simulink model "APA_AEB_Version_0_1"  (R2019a)
settings: Solver=FixedStepAuto  StartTime=0.0  StopTime=2  FixedStep=0.01  RelTol=1e-3
libraries: simulink x4, dspnetwork x1, autolibshared x1
(part 1 of 3)
settings Model: DataDictionary=AEB_APA_V1.sldd  EnableAccessToBaseWorkspace=off  Creator=root  LastModifiedBy=wz527
settings DataIOCC: ReturnWorkspaceOutputs=off
settings OptimizationCC: UseDivisionForNetSlopeComputation=on  DefaultUnderspecifiedDataType=single
settings DebuggingCC: ArithmeticOperatorsInVariantConditions=warning

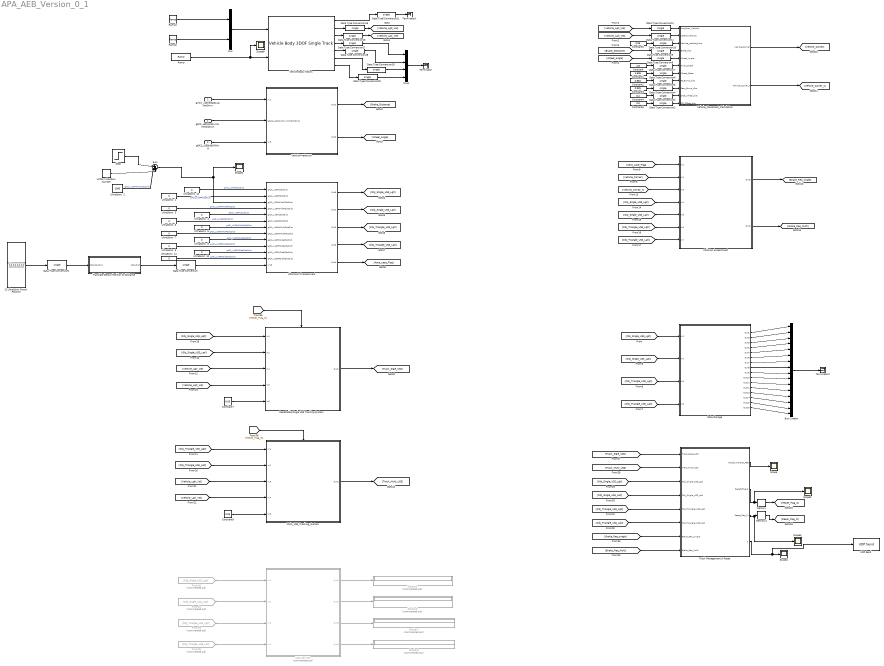
== system APA_AEB_Version_0_1 ==
  gSCS_u8RNonDrvnWhlRotlDircn : Inport
  gVCU_u16VelSpdAvgNonDrvn : Inport  Port=2
  gSAS_u16StrgWhlAng : Inport  Port=3
  12 UltraSonic Mount Position : Constant  Value=[1 1;0 0;0 0;0 0;0 0;0 0;0 0;0 0;0 0;0 0;0 0;0 0]  VectorParams1D=off
  Bus Creator : BusCreator  Inputs=16
  Collision Assessment : Subsystem
  Constant : Constant  Value=2.8
  Constant1 : Constant  Value=1.606
  Constant2 : Constant  Value=0.953
  Constant3 : Constant  Value=0.925
  Constant4 : Constant  Value=0.2
  Constant5 : Constant  Value=0.05
  Constant6 : Constant  Value=0.5
  Constant7 : Constant  Value=0.05  OutDataTypeStr=single
  Constant9 : Constant  Value=0.05  OutDataTypeStr=single
  Data Storage : Subsystem
  Data Type Conversion{,1..12,15..21} (20 alike) : DataTypeConversion  OutDataTypeStr=single
  Display{5..8} (4 alike) : Display  Commented=on
  From23 : From  Commented=on  GotoTag=Obj_Triangle_USS_Lgtl
  From24 : From  Commented=on  GotoTag=Obj_Single_USS_Latl
  From25 : From  Commented=on  GotoTag=Obj_Triangle_USS_Latl
  From26 : From  Commented=on  GotoTag=Obj_Single_USS_Lgtl
  Memory : Memory
  Memory1 : Memory
  Multi_USS_Tracking_System : Subsystem
  Mux : Mux  Inputs=2
  Mux1 : Mux
  Ramp : simulink/Sources/Ramp  slope=0.1  start=0  InitialOutput=5
  Ramp1 : simulink/Sources/Ramp  slope=1  start=0  InitialOutput=0
  Ramp2 : simulink/Sources/Ramp  slope=1  start=0  InitialOutput=0
  Resettable Single USS Tracking System : Subsystem  TreatAsAtomicUnit=on
  Scope{,1..4,9} (6 alike) : Scope
  Step : Step  After=300  SampleTime=0
  Sum : Sum  Inputs=|+++
  Terminator : Terminator
  Terminator1 : Terminator
  Terminator2 : Terminator
  Track Management & Reset : MATLAB Function  TreatAsAtomicUnit=on
  Translate Sensor Position to Distance : MATLAB Function  TreatAsAtomicUnit=on
  UDP Send : dspnetwork/UDP Send  remoteURL='192.168.101.1'  remotePort=12  localURL='0.0.0.0'  localPortSource=Automatically determine  localPort=-1  sampletime=-1  blockPlatform=[]  separateLengthPort=0
      settings: SourceProductName=Simulink
  USS Wall HMI : Subsystem  Commented=on
  "Ultarsonic Processment " : Subsystem  Tag=USS_Module  VariantControlMode=Label  Variant=on  VariantControl=Variant1  LabelModeActiveChoice=Variant1
  UltraSonic  {1,3..12} (11 alike) : Constant  Value=0  VectorParams1D=off  SampleTime=0.1
  UltraSonic  2 : Constant  Value=1000  VectorParams1D=off  SampleTime=0.1
  Uniform Random Number : UniformRandomNumber  Minimum=-100  Maximum=50  SampleTime=0.01
  Vehicle Body Motion : autolibshared/Vehicle Body 3DOF Single Track  trackMode=Dual  inputMode=External longitudinal velocity  frontSteerMode=on  rearSteerMode=off  windMode=off  muMode=off  extFMode=off  extMMode=off  extXo=off  extpsio=off  extxdoto=off  extro=off  extYo=off  extTamb=off  extydoto=off  aMode=2  NF=2  NR=2  m=2000  a=1.4  b=1.6  h=0.35  X_o=0  xdot_o=0  CalphaMode=off  sigmaMode=on  d=0  w=[1.4,1.4]  Cy_f=12e3  Cy_r=11e3  sigma_f=.1  sigma_r=.1  alpha_f_brk=[-.1 .1]  Cy_f_data=[-9e3 9e3]  alpha_r_brk=[-.1 .1]  Cy_r_data=[-9e3 9e3]  Y_o=0  ydot_o=0  Izz=4000  psi_o=0  r_o=0  Af=2  Cd=.3  Cl=.1  Cpm=.1  beta_w=[0:0.01:0.3]  Cs=[0:0.03:0.9]  Cym=[0:0.01:0.3]  Pabs=101325  Tair=273  g=9.81  mu=1  xdot_tol=.01  Fznom=5000  Fxtire_sat=7e4  Fytire_sat=7e4  longOff=0  latOff=0  vertOff=0  wrapAng=off
      settings: SourceProductName=Powertrain Blockset  SourceProductBaseCode=PW
  Vehicle Prediction : Subsystem
  Vehicle_Movement_Calculation : MATLAB Function  TreatAsAtomicUnit=on
  wires:
  gVCU_u16VelSpdAvgNonDrvn/1 -> Vehicle Prediction/1(In1)
  gSCS_u8RNonDrvnWhlRotlDircn/1 -> Vehicle Prediction/2(gSCS_u8RNonDrvnWhlRotlDircn)
  gSAS_u16StrgWhlAng/1 -> Vehicle Prediction/3(In3)
  12 UltraSonic Mount Position/1 -> Data Type Conversion1/1
  UltraSonic  12/1 -> "Ultarsonic Processment "/1(gASI_u16FLObsDist)  "gASI_u16FLObsDist"
  Vehicle Body Motion/1 -> Data Type Conversion21/1
  Vehicle Body Motion/4 -> Data Type Conversion17/1
  Vehicle Body Motion/6 -> Data Type Conversion19/1
  Vehicle Body Motion/7 -> Data Type Conversion20/1
  Vehicle Body Motion/5 -> Data Type Conversion18/1
  Mux1/1 -> Terminator/1
  Constant/1 -> Data Type Conversion7/1
  Constant1/1 -> Data Type Conversion6/1
  Constant2/1 -> Data Type Conversion5/1
  Constant3/1 -> Data Type Conversion4/1
  Constant4/1 -> Data Type Conversion3/1
  Constant5/1 -> Data Type Conversion10/1
  Constant6/1 -> Data Type Conversion2/1
  Vehicle Body Motion/2 -> Data Type Conversion15/1
  Vehicle Body Motion/3 -> Data Type Conversion16/1
  [Vehicle_Lgtl_Vel] -> Data Type Conversion12/1
  [Vehicle_Latl_Vel] -> Data Type Conversion11/1
  Vehicle Prediction/1(Out1) -> [Brake_Distance]
  Vehicle Prediction/2(Out2) -> [Wheel_Angle]
  [Brake_Distance] -> Data Type Conversion9/1
  [Wheel_Angle] -> Data Type Conversion8/1
  UltraSonic  1/1 -> "Ultarsonic Processment "/2(gASI_u16FRObsDist)  "gASI_u16FRObsDist"
  UltraSonic  3/1 -> "Ultarsonic Processment "/4(gASI_u16FrtMidRObsDist)  "gASI_u16FrtMidRObsDist"
  UltraSonic  4/1 -> "Ultarsonic Processment "/5(gASI_u16RLObsDist)  "gASI_u16RLObsDist"
  UltraSonic  5/1 -> "Ultarsonic Processment "/6(gASI_u16RRObsDist)  "gASI_u16RRObsDist"
  UltraSonic  6/1 -> "Ultarsonic Processment "/7(gASI_u16RrtMidLObsDist)  "gASI_u16RrtMidLObsDist"
  UltraSonic  7/1 -> "Ultarsonic Processment "/8(gASI_u16RrtMidRObsDist)  "gASI_u16RrtMidRObsDist"
  UltraSonic  8/1 -> "Ultarsonic Processment "/9(gASI_u16FLSideObsDist)  "gASI_u16FLSideObsDist"
  UltraSonic  9/1 -> "Ultarsonic Processment "/10(gASI_u16FRSideObsDist)  "gASI_u16FRSideObsDist"
  UltraSonic  10/1 -> "Ultarsonic Processment "/11(gASI_u16RLSideObsDist)  "gASI_u16RLSideObsDist"
  UltraSonic  11/1 -> "Ultarsonic Processment "/12(gASI_u16RRSideObsDist)  "gASI_u16RRSideObsDist"
  Translate Sensor Position to Distance/1(USS_Dist) -> Data Type Conversion/1
  "Ultarsonic Processment "/1(Out6) -> [Obj_Single_USS_Lgtl]
  "Ultarsonic Processment "/2(Out1) -> [Obj_Single_USS_Latl]
  "Ultarsonic Processment "/3(Out2) -> [Obj_Triangle_USS_Lgtl]
  "Ultarsonic Processment "/4(Out3) -> [Obj_Triangle_USS_Latl]
  Vehicle_Movement_Calculation/1(Vehicle_Corner) -> [Vehicle_Corner]
  Vehicle_Movement_Calculation/2(Vehicle_Corner_t) -> [Vehicle_Corner_t]
  [Obj_Single_USS_Lgtl] -> Data Storage/1(In2)
  [Obj_Single_USS_Latl] -> Data Storage/2(In4)
  [Obj_Triangle_USS_Lgtl] -> Data Storage/3(In5)
  [Obj_Triangle_USS_Latl] -> Data Storage/4(In6)
  "Ultarsonic Processment "/5(Out4) -> [Aera_case_Flag]
  [Aera_case_Flag] -> Collision Assessment/1(In1)
  [Vehicle_Corner] -> Collision Assessment/2(In2)
  [Vehicle_Corner_t] -> Collision Assessment/3(In3)
  [Obj_Single_USS_Lgtl] -> Collision Assessment/4(In4)
  [Obj_Single_USS_Latl] -> Collision Assessment/5(In5)
  [Obj_Triangle_USS_Lgtl] -> Collision Assessment/6(In6)
  [Obj_Triangle_USS_Latl] -> Collision Assessment/7(In7)
  Data Storage/1(Out1) -> Bus Creator/1
  Data Storage/2(Out3) -> Bus Creator/2
  Data Storage/3(Out5) -> Bus Creator/3
  Data Storage/4(Out2) -> Bus Creator/4
  Data Storage/5(Out4) -> Bus Creator/5
  Data Storage/6(Out6) -> Bus Creator/6
  Data Storage/7(Out7) -> Bus Creator/7
  Data Storage/8(Out8) -> Bus Creator/8
  Data Storage/9(Out9) -> Bus Creator/9
  Data Storage/10(Out10) -> Bus Creator/10
  Data Storage/11(Out11) -> Bus Creator/11
  Data Storage/12(Out12) -> Bus Creator/12
  Data Storage/13(Out13) -> Bus Creator/13
  Data Storage/14(Out14) -> Bus Creator/14
  Data Storage/15(Out15) -> Bus Creator/15
  Data Storage/16(Out16) -> Bus Creator/16
  Bus Creator/1 -> Terminator2/1
  [Obj_Single_USS_Lgtl] -> Resettable Single USS Tracking System/1(In1)
  [Obj_Single_USS_Latl] -> Resettable Single USS Tracking System/2(In2)
  [Vehicle_Lgtl_Vel] -> Resettable Single USS Tracking System/3(In4)
  [Vehicle_Latl_Vel] -> Resettable Single USS Tracking System/4(In5)
  Constant7/1 -> Resettable Single USS Tracking System/5(In6)
  Resettable Single USS Tracking System/1(Out1) -> [Track_Sigle_USS]
  Collision Assessment/1(Out3) -> [Brake_Req_single]
  Collision Assessment/2(Out1) -> [Brake_Req_Multi]
  UltraSonic  2/1 -> Sum/2  "gASI_u16FrtMidLObsDist"
  Sum/1 -> "Ultarsonic Processment "/3(gASI_u16FrtMidLObsDist), Scope1/1
  [Obj_Triangle_USS_Lgtl] -> Multi_USS_Tracking_System/1(In1)
  [Obj_Triangle_USS_Latl] -> Multi_USS_Tracking_System/2(In2)
  [Vehicle_Lgtl_Vel] -> Multi_USS_Tracking_System/3(In3)
  [Vehicle_Latl_Vel] -> Multi_USS_Tracking_System/4(In4)
  Constant9/1 -> Multi_USS_Tracking_System/5(In5)
  Multi_USS_Tracking_System/1(Out1) -> [Track_Multi_USS]
  From26/1 -> USS Wall HMI/1(In1)
  From24/1 -> USS Wall HMI/2(In2)
  From23/1 -> USS Wall HMI/3(In3)
  From25/1 -> USS Wall HMI/4(In4)
  USS Wall HMI/1(Out1) -> Display5/1
  USS Wall HMI/2(Out2) -> Display6/1
  USS Wall HMI/3(Out3) -> Display7/1
  USS Wall HMI/4(Out4) -> Display8/1
  [Track_Sigle_USS] -> Track Management & Reset/1(Track_Sigle_USS)
  [Track_Multi_USS] -> Track Management & Reset/2(Track_Multi_USS)
  [Obj_Single_USS_Lgtl] -> Track Management & Reset/3(Obj_Single_USS_Lgtl)
  [Obj_Single_USS_Latl] -> Track Management & Reset/4(Obj_Single_USS_Latl)
  [Obj_Triangle_USS_Lgtl] -> Track Management & Reset/5(Obj_Triangle_USS_Lgtl)
  [Obj_Triangle_USS_Latl] -> Track Management & Reset/6(Obj_Triangle_USS_Latl)
  [Brake_Req_single] -> Track Management & Reset/7(Brake_Req_single)
  [Brake_Req_Multi] -> Track Management & Reset/8(Brake_Req_Multi)
  Step/1 -> Sum/1
  Uniform Random Number/1 -> Sum/3
  Track Management & Reset/1(Global_Tracker_AEB) -> Scope/1
  Track Management & Reset/2(Reset_Flag_S) -> Scope2/1, Memory/1
  Track Management & Reset/3(Reset_Flag_M) -> Scope3/1, Memory1/1
  [Reset_Flag_S] -> Resettable Single USS Tracking System/Reset
  [Reset_Flag_M] -> Multi_USS_Tracking_System/Reset
  Memory/1 -> [Reset_Flag_S]
  Memory1/1 -> [Reset_Flag_M]
  Track Management & Reset/4(c) -> UDP Send/1, Scope4/1
  Data Type Conversion/1 -> "Ultarsonic Processment "/13(In13)
  Data Type Conversion1/1 -> Translate Sensor Position to Distance/1(USS_Position)
  Data Type Conversion2/1 -> Vehicle_Movement_Calculation/11(CG_Offset_dist)
  Data Type Conversion3/1 -> Vehicle_Movement_Calculation/10(Side_wheel_dist)
  Data Type Conversion4/1 -> Vehicle_Movement_Calculation/9(Rear_Bump_dist)
  Data Type Conversion5/1 -> Vehicle_Movement_Calculation/8(Frt_Bump_dist)
  Data Type Conversion6/1 -> Vehicle_Movement_Calculation/7(Wheel_Base)
  Data Type Conversion7/1 -> Vehicle_Movement_Calculation/6(Axle_Length)
  Data Type Conversion8/1 -> Vehicle_Movement_Calculation/5(Wheel_Angle)
  Data Type Conversion9/1 -> Vehicle_Movement_Calculation/4(Brake_dist)
  Data Type Conversion10/1 -> Vehicle_Movement_Calculation/3(Vehicle_predict_time)
  Data Type Conversion11/1 -> Vehicle_Movement_Calculation/2(Lateral_Velocity)
  Data Type Conversion12/1 -> Vehicle_Movement_Calculation/1(Longitual_Velocity)
  Mux/1 -> Vehicle Body Motion/1
  Data Type Conversion15/1 -> [Vehicle_Lgtl_Vel]
  Data Type Conversion16/1 -> [Vehicle_Latl_Vel]
  Data Type Conversion17/1 -> Mux1/1
  Data Type Conversion18/1 -> Mux1/2
  Data Type Conversion19/1 -> Mux1/3
  Data Type Conversion20/1 -> Mux1/4
  Data Type Conversion21/1 -> Terminator1/1
  Ramp1/1 -> Mux/1
  Ramp2/1 -> Mux/2
  Ramp/1 -> Scope9/1, Vehicle Body Motion/2

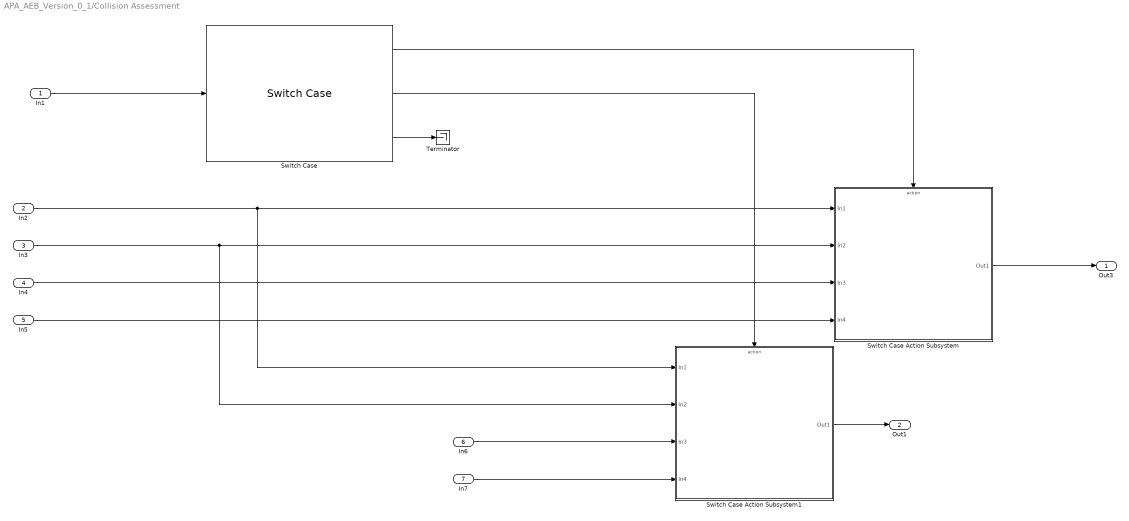
== system APA_AEB_Version_0_1/Collision Assessment ==
  In1 : Inport
  In2 : Inport  Port=2
  In3 : Inport  Port=3
  In4 : Inport  Port=4
  In5 : Inport  Port=5
  In6 : Inport  Port=6
  In7 : Inport  Port=7
  Switch Case : SwitchCase  CaseConditions={[1,2,3,4,5,6,7,8,9,10,11,12],[14,15,16,20,21,22]}
  Switch Case Action Subsystem : Subsystem  TreatAsAtomicUnit=on
  Switch Case Action Subsystem1 : Subsystem  TreatAsAtomicUnit=on
  Terminator : Terminator
  Out3 : Outport
  Out1 : Outport  Port=2
  wires:
  Switch Case Action Subsystem/1(Out1) -> Out3/1
  Switch Case/2 -> Switch Case Action Subsystem1/Action
  In1/1 -> Switch Case/1
  In2/1 -> Switch Case Action Subsystem1/1(In1), Switch Case Action Subsystem/1(In1)
  In4/1 -> Switch Case Action Subsystem/3(In3)
  In3/1 -> Switch Case Action Subsystem1/2(In2), Switch Case Action Subsystem/2(In2)
  Switch Case/3 -> Terminator/1
  In5/1 -> Switch Case Action Subsystem/4(In4)
  Switch Case/1 -> Switch Case Action Subsystem/Action
  In6/1 -> Switch Case Action Subsystem1/3(In3)
  In7/1 -> Switch Case Action Subsystem1/4(In4)
  Switch Case Action Subsystem1/1(Out1) -> Out1/1

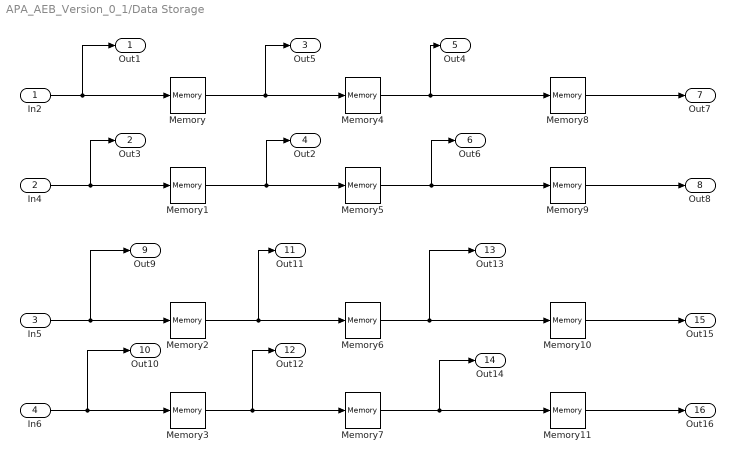
== system APA_AEB_Version_0_1/Data Storage ==
  In2 : Inport
  In4 : Inport  Port=2
  In5 : Inport  Port=3
  In6 : Inport  Port=4
  Memory{,1..11} (12 alike) : Memory
  Out1 : Outport
  Out3 : Outport  Port=2
  Out5 : Outport  Port=3
  Out2 : Outport  Port=4
  Out4 : Outport  Port=5
  Out6 : Outport  Port=6
  Out7 : Outport  Port=7
  Out8 : Outport  Port=8
  Out9 : Outport  Port=9
  Out10 : Outport  Port=10
  Out11 : Outport  Port=11
  Out12 : Outport  Port=12
  Out13 : Outport  Port=13
  Out14 : Outport  Port=14
  Out15 : Outport  Port=15
  Out16 : Outport  Port=16
  wires:
  Memory3/1 -> Out12/1, Memory7/1
  Memory2/1 -> Out11/1, Memory6/1
  Memory7/1 -> Out14/1, Memory11/1
  Memory6/1 -> Out13/1, Memory10/1
  In5/1 -> Out9/1, Memory2/1
  In4/1 -> Out3/1, Memory1/1
  Memory/1 -> Out5/1, Memory4/1
  Memory1/1 -> Memory5/1, Out2/1
  In6/1 -> Out10/1, Memory3/1
  Memory4/1 -> Out4/1, Memory8/1
  Memory5/1 -> Memory9/1, Out6/1
  Memory8/1 -> Out7/1
  Memory9/1 -> Out8/1
  In2/1 -> Out1/1, Memory/1
  Memory10/1 -> Out15/1
  Memory11/1 -> Out16/1

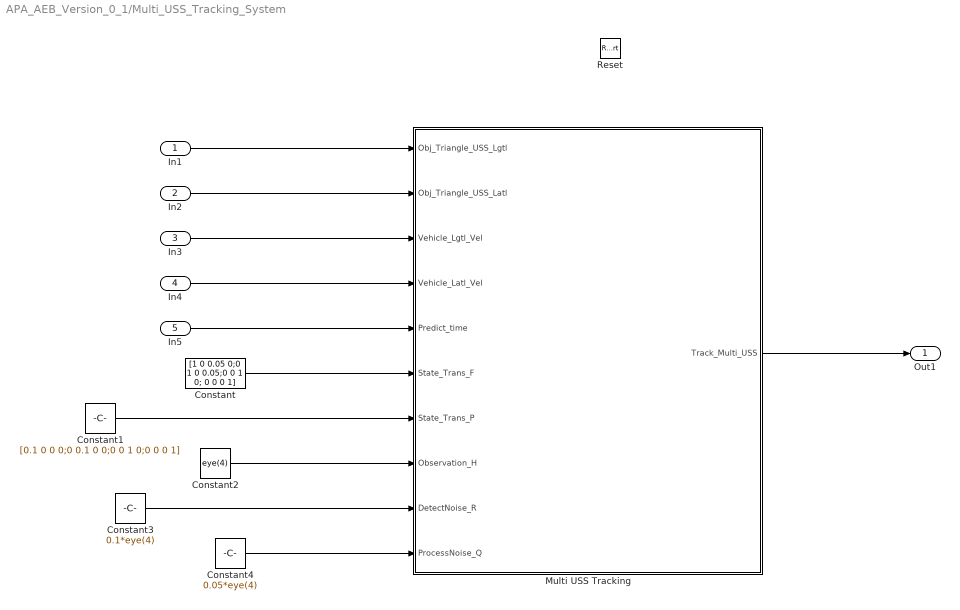
== system APA_AEB_Version_0_1/Multi_USS_Tracking_System ==
  In1 : Inport
  In2 : Inport  Port=2
  In3 : Inport  Port=3
  In4 : Inport  Port=4
  In5 : Inport  Port=5
  Reset : ResetPort  DisableCoverage=on  ResetTriggerType=level hold
  Constant : Constant  Value=[1 0 0.05 0;0 1 0 0.05;0 0 1 0; 0 0 0 1]  OutDataTypeStr=single
  Constant1 : Constant  Value=[0.1 0 0 0;0 0.1 0 0;0 0 1 0;0 0 0 1]  OutDataTypeStr=single
  Constant2 : Constant  Value=eye(4)  OutDataTypeStr=single
  Constant3 : Constant  Value=0.1*eye(4)  OutDataTypeStr=single
  Constant4 : Constant  Value=0.05*eye(4)  OutDataTypeStr=single
  Multi USS Tracking : MATLAB Function  TreatAsAtomicUnit=on
  Out1 : Outport
  wires:
  In4/1 -> Multi USS Tracking/4(Vehicle_Latl_Vel)
  Multi USS Tracking/1(Track_Multi_USS) -> Out1/1
  Constant4/1 -> Multi USS Tracking/10(ProcessNoise_Q)
  In5/1 -> Multi USS Tracking/5(Predict_time)
  Constant1/1 -> Multi USS Tracking/7(State_Trans_P)
  Constant2/1 -> Multi USS Tracking/8(Observation_H)
  Constant/1 -> Multi USS Tracking/6(State_Trans_F)
  In3/1 -> Multi USS Tracking/3(Vehicle_Lgtl_Vel)
  Constant3/1 -> Multi USS Tracking/9(DetectNoise_R)
  In1/1 -> Multi USS Tracking/1(Obj_Triangle_USS_Lgtl)
  In2/1 -> Multi USS Tracking/2(Obj_Triangle_USS_Latl)

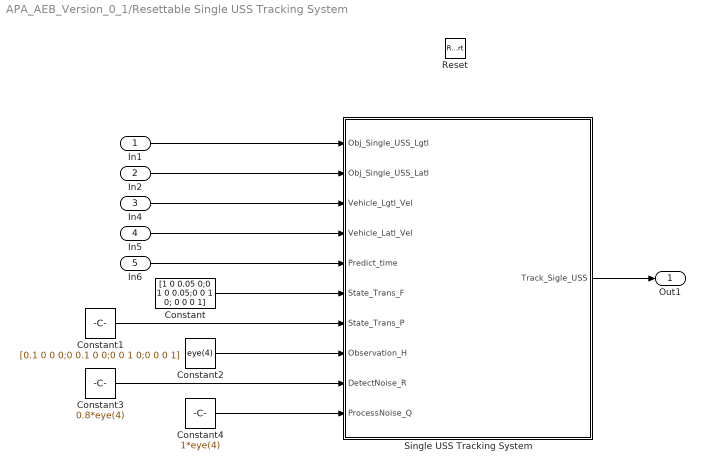
== system APA_AEB_Version_0_1/Resettable Single USS Tracking System ==
  In1 : Inport
  In2 : Inport  Port=2
  In4 : Inport  Port=3
  In5 : Inport  Port=4
  In6 : Inport  Port=5
  Reset : ResetPort  DisableCoverage=on  ResetTriggerType=level hold
  Constant : Constant  Value=[1 0 0.05 0;0 1 0 0.05;0 0 1 0; 0 0 0 1]  OutDataTypeStr=single
  Constant1 : Constant  Value=[0.1 0 0 0;0 0.1 0 0;0 0 1 0;0 0 0 1]  OutDataTypeStr=single
  Constant2 : Constant  Value=eye(4)  OutDataTypeStr=single
  Constant3 : Constant  Value=0.8*eye(4)  OutDataTypeStr=single
  Constant4 : Constant  Value=1*eye(4)  OutDataTypeStr=single
  Single USS Tracking System : MATLAB Function  TreatAsAtomicUnit=on
  Out1 : Outport
  wires:
  Single USS Tracking System/1(Track_Sigle_USS) -> Out1/1
  In1/1 -> Single USS Tracking System/1(Obj_Single_USS_Lgtl)
  In4/1 -> Single USS Tracking System/3(Vehicle_Lgtl_Vel)
  In5/1 -> Single USS Tracking System/4(Vehicle_Latl_Vel)
  In2/1 -> Single USS Tracking System/2(Obj_Single_USS_Latl)
  In6/1 -> Single USS Tracking System/5(Predict_time)
  Constant/1 -> Single USS Tracking System/6(State_Trans_F)
  Constant1/1 -> Single USS Tracking System/7(State_Trans_P)
  Constant2/1 -> Single USS Tracking System/8(Observation_H)
  Constant3/1 -> Single USS Tracking System/9(DetectNoise_R)
  Constant4/1 -> Single USS Tracking System/10(ProcessNoise_Q)

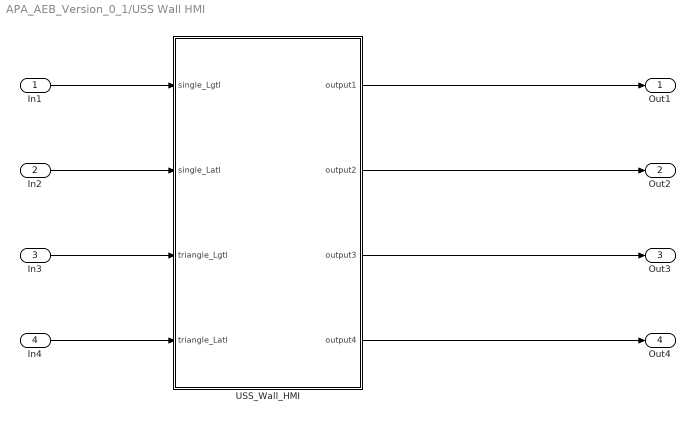
== system APA_AEB_Version_0_1/USS Wall HMI ==
  In1 : Inport
  In2 : Inport  Port=2
  In3 : Inport  Port=3
  In4 : Inport  Port=4
  USS_Wall_HMI : MATLAB Function  TreatAsAtomicUnit=on
  Out1 : Outport
  Out2 : Outport  Port=2
  Out3 : Outport  Port=3
  Out4 : Outport  Port=4
  wires:
  In2/1 -> USS_Wall_HMI/2(single_Latl)
  USS_Wall_HMI/1(output1) -> Out1/1
  In3/1 -> USS_Wall_HMI/3(triangle_Lgtl)
  USS_Wall_HMI/2(output2) -> Out2/1
  USS_Wall_HMI/3(output3) -> Out3/1
  In1/1 -> USS_Wall_HMI/1(single_Lgtl)
  In4/1 -> USS_Wall_HMI/4(triangle_Latl)
  USS_Wall_HMI/4(output4) -> Out4/1

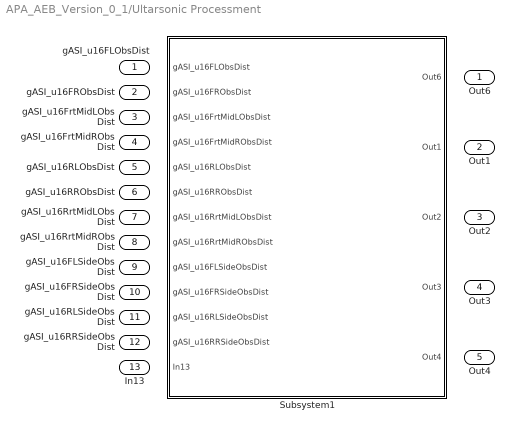
== system APA_AEB_Version_0_1/Ultarsonic Processment  ==
  gASI_u16FLObsDist : Inport
  gASI_u16FRObsDist : Inport  Port=2
  gASI_u16FrtMidLObsDist : Inport  Port=3
  gASI_u16FrtMidRObsDist : Inport  Port=4
  gASI_u16RLObsDist : Inport  Port=5
  gASI_u16RRObsDist : Inport  Port=6
  gASI_u16RrtMidLObsDist : Inport  Port=7
  gASI_u16RrtMidRObsDist : Inport  Port=8
  gASI_u16FLSideObsDist : Inport  Port=9
  gASI_u16FRSideObsDist : Inport  Port=10
  gASI_u16RLSideObsDist : Inport  Port=11
  gASI_u16RRSideObsDist : Inport  Port=12
  In13 : Inport  Port=13
  Subsystem1 : Subsystem  VariantControlMode=Label  Variant=on  VariantControl=Variant1  LabelModeActiveChoice=Variant1
  Out6 : Outport
  Out1 : Outport  Port=2
  Out2 : Outport  Port=3
  Out3 : Outport  Port=4
  Out4 : Outport  Port=5

== system APA_AEB_Version_0_1/Vehicle Prediction ==
  In1 : Inport
  gSCS_u8RNonDrvnWhlRotlDircn : Inport  Port=2
  In3 : Inport  Port=3
  Subsystem : Subsystem
  Subsystem1 : Subsystem
  Out1 : Outport
  Out2 : Outport  Port=2
  wires:
  In1/1 -> Subsystem/1(In1)
  gSCS_u8RNonDrvnWhlRotlDircn/1 -> Subsystem/2(gSCS_u8RNonDrvnWhlRotlDircn)
  Subsystem/1(Out1) -> Out1/1
  In3/1 -> Subsystem1/1(In1)
  Subsystem1/1(Out1) -> Out2/1

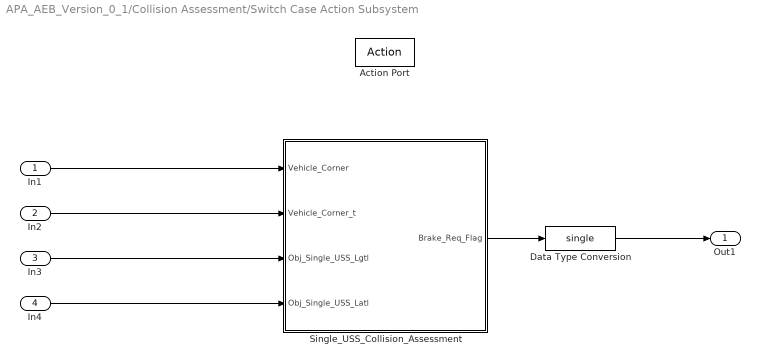
== system APA_AEB_Version_0_1/Collision Assessment/Switch Case Action Subsystem ==
  In1 : Inport
  In2 : Inport  Port=2
  In3 : Inport  Port=3
  In4 : Inport  Port=4
  Action Port : ActionPort  ActionPortLabel=case [ 1 2 3 4 5 6 7 8 9 10 11 12 ]:
  Data Type Conversion : DataTypeConversion  OutDataTypeStr=single
  Single_USS_Collision_Assessment : MATLAB Function  TreatAsAtomicUnit=on
  Out1 : Outport
  wires:
  In1/1 -> Single_USS_Collision_Assessment/1(Vehicle_Corner)
  In2/1 -> Single_USS_Collision_Assessment/2(Vehicle_Corner_t)
  In3/1 -> Single_USS_Collision_Assessment/3(Obj_Single_USS_Lgtl)
  In4/1 -> Single_USS_Collision_Assessment/4(Obj_Single_USS_Latl)
  Single_USS_Collision_Assessment/1(Brake_Req_Flag) -> Data Type Conversion/1
  Data Type Conversion/1 -> Out1/1

== system APA_AEB_Version_0_1/Collision Assessment/Switch Case Action Subsystem1 ==
  In1 : Inport
  In2 : Inport  Port=2
  In3 : Inport  Port=3
  In4 : Inport  Port=4
  Action Port : ActionPort  ActionPortLabel=case [ 14 15 16 20 21 22 ]:
  Multi_USS_Collision_Assessment : MATLAB Function  TreatAsAtomicUnit=on
  Out1 : Outport
  wires:
  Multi_USS_Collision_Assessment/1(Brake_Req_Flag) -> Out1/1
  In4/1 -> Multi_USS_Collision_Assessment/4(Obj_Triangle_USS_Latl)
  In3/1 -> Multi_USS_Collision_Assessment/3(Obj_Triangle_USS_Lgtl)
  In2/1 -> Multi_USS_Collision_Assessment/2(Vehicle_Corner_t)
  In1/1 -> Multi_USS_Collision_Assessment/1(Vehicle_Corner)

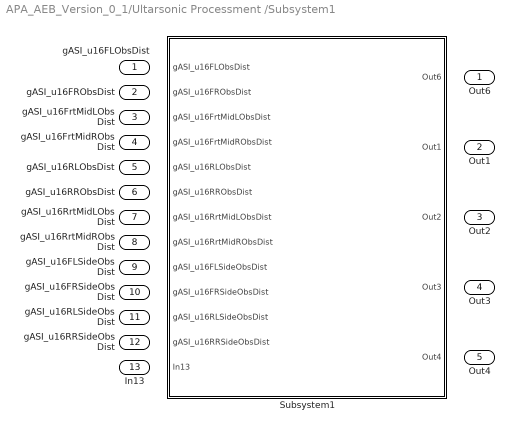
== system APA_AEB_Version_0_1/Ultarsonic Processment /Subsystem1 ==
  gASI_u16FLObsDist : Inport
  gASI_u16FRObsDist : Inport  Port=2
  gASI_u16FrtMidLObsDist : Inport  Port=3
  gASI_u16FrtMidRObsDist : Inport  Port=4
  gASI_u16RLObsDist : Inport  Port=5
  gASI_u16RRObsDist : Inport  Port=6
  gASI_u16RrtMidLObsDist : Inport  Port=7
  gASI_u16RrtMidRObsDist : Inport  Port=8
  gASI_u16FLSideObsDist : Inport  Port=9
  gASI_u16FRSideObsDist : Inport  Port=10
  gASI_u16RLSideObsDist : Inport  Port=11
  gASI_u16RRSideObsDist : Inport  Port=12
  In13 : Inport  Port=13
  Subsystem1 : Subsystem  VariantControl=Variant1
  Out6 : Outport
  Out1 : Outport  Port=2
  Out2 : Outport  Port=3
  Out3 : Outport  Port=4
  Out4 : Outport  Port=5

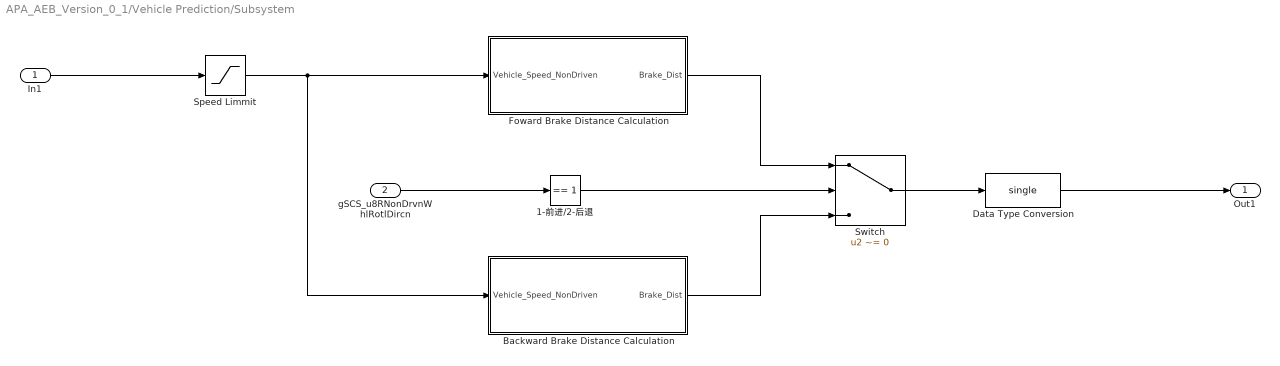
== system APA_AEB_Version_0_1/Vehicle Prediction/Subsystem ==
  In1 : Inport
  gSCS_u8RNonDrvnWhlRotlDircn : Inport  Port=2
  1-前进/2-后退 : simulink/Logic and Bit Operations/Compare To Constant  relop===  const=1  OutDataTypeStr=boolean
  Backward Brake Distance Calculation : MATLAB Function  TreatAsAtomicUnit=on
  Data Type Conversion : DataTypeConversion  OutDataTypeStr=single
  Foward Brake Distance Calculation : MATLAB Function  TreatAsAtomicUnit=on
  Speed Limmit : Saturate  UpperLimit=6  LowerLimit=0
  Switch : Switch  Criteria=u2 ~= 0
  Out1 : Outport
  wires:
  Backward Brake Distance Calculation/1(Brake_Dist) -> Switch/3
  Speed Limmit/1 -> Backward Brake Distance Calculation/1(Vehicle_Speed_NonDriven), Foward Brake Distance Calculation/1(Vehicle_Speed_NonDriven)
  Data Type Conversion/1 -> Out1/1
  Foward Brake Distance Calculation/1(Brake_Dist) -> Switch/1
  1-前进/2-后退/1 -> Switch/2
  Switch/1 -> Data Type Conversion/1
  gSCS_u8RNonDrvnWhlRotlDircn/1 -> 1-前进/2-后退/1
  In1/1 -> Speed Limmit/1

== system APA_AEB_Version_0_1/Vehicle Prediction/Subsystem1 ==
  In1 : Inport
  Data Type Conversion1 : DataTypeConversion  OutDataTypeStr=single
  Data Type Conversion3 : DataTypeConversion  OutDataTypeStr=single
  Steer Angle To Wheel Angle : MATLAB Function  TreatAsAtomicUnit=on
  Out1 : Outport
  wires:
  Data Type Conversion3/1 -> Steer Angle To Wheel Angle/1(Steer_Angle)
  Steer Angle To Wheel Angle/1(Wheel_Angle) -> Data Type Conversion1/1
  In1/1 -> Data Type Conversion3/1
  Data Type Conversion1/1 -> Out1/1

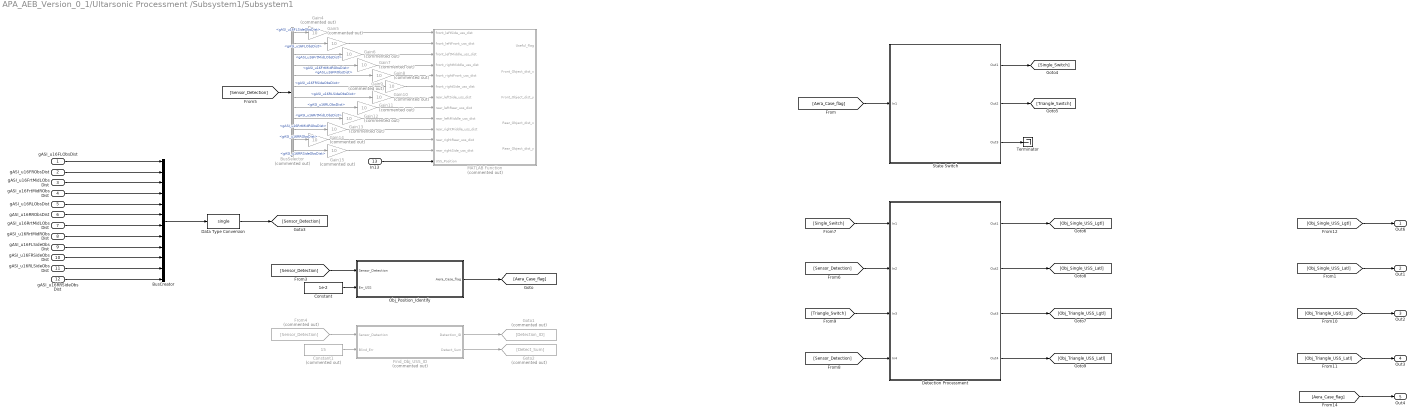
== system APA_AEB_Version_0_1/Ultarsonic Processment /Subsystem1/Subsystem1 ==
  gASI_u16FLObsDist : Inport
  gASI_u16FRObsDist : Inport  Port=2
  gASI_u16FrtMidLObsDist : Inport  Port=3
  gASI_u16FrtMidRObsDist : Inport  Port=4
  gASI_u16RLObsDist : Inport  Port=5
  gASI_u16RRObsDist : Inport  Port=6
  gASI_u16RrtMidLObsDist : Inport  Port=7
  gASI_u16RrtMidRObsDist : Inport  Port=8
  gASI_u16FLSideObsDist : Inport  Port=9
  gASI_u16FRSideObsDist : Inport  Port=10
  gASI_u16RLSideObsDist : Inport  Port=11
  gASI_u16RRSideObsDist : Inport  Port=12
  In13 : Inport  Port=13
  BusCreator : BusCreator  Inputs=12
  BusSelector : BusSelector  Commented=on  OutputSignals=gASI_u16FLSideObsDist,gASI_u16FLObsDist,gASI_u16FrtMidLObsDist,gASI_u16FrtMidRObsDist,gASI_u16FRObsDist,gASI_u16FRSideObsDist,gASI_u16RLSideObsDist,gASI_u16RLObsDist,gASI_u16RrtMidLObsDist,gASI_u16RrtMidRObsDist,gASI_u16RRObsDist,gASI_u16RRSideObsDist
  Constant : Constant  Value=1e-2  OutDataTypeStr=single
  Constant1 : Constant  Commented=on  Value=15
  Data Type Conversion : DataTypeConversion  OutDataTypeStr=single
  Detection Processment : Subsystem
  Find_Obj_USS_ID : MATLAB Function  Commented=on  TreatAsAtomicUnit=on
  From4 : From  Commented=on  GotoTag=Sensor_Detection
  Gain{4..15} (12 alike) : Gain  Commented=on  Gain=10  OutDataTypeStr=Inherit: Same as input
  Goto1 : Goto  Commented=on  GotoTag=Detection_ID
  Goto2 : Goto  Commented=on  GotoTag=Detect_Sum
  MATLAB Function : MATLAB Function  Commented=on  TreatAsAtomicUnit=on
  Obj_Position_Identify : MATLAB Function  TreatAsAtomicUnit=on
  State Switch : Subsystem
  Terminator : Terminator
  Out6 : Outport
  Out1 : Outport  Port=2
  Out2 : Outport  Port=3
  Out3 : Outport  Port=4
  Out4 : Outport  Port=5
  wires:
  BusSelector/5 -> Gain8/1  "<gASI_u16FRObsDist>"
  BusCreator/1 -> Data Type Conversion/1
  BusSelector/1 -> Gain4/1  "<gASI_u16FLSideObsDist>"
  gASI_u16RRObsDist/1 -> BusCreator/6
  BusSelector/10 -> Gain13/1  "<gASI_u16RrtMidRObsDist>"
  BusSelector/4 -> Gain7/1  "<gASI_u16FrtMidRObsDist>"
  Gain13/1 -> MATLAB Function/10(rear_rightMiddle_uss_dist)
  BusSelector/3 -> Gain6/1  "<gASI_u16FrtMidLObsDist>"
  BusSelector/11 -> Gain14/1  "<gASI_u16RRObsDist>"
  gASI_u16FRSideObsDist/1 -> BusCreator/10
  BusSelector/12 -> Gain15/1  "<gASI_u16RRSideObsDist>"
  Gain9/1 -> MATLAB Function/6(front_rightSide_uss_dist)
  Gain10/1 -> MATLAB Function/7(rear_leftSide_uss_dist)
  BusSelector/8 -> Gain11/1  "<gASI_u16RLObsDist>"
  Gain7/1 -> MATLAB Function/4(front_rightMiddle_uss_dist)
  BusSelector/6 -> Gain9/1  "<gASI_u16FRSideObsDist>"
  gASI_u16FrtMidRObsDist/1 -> BusCreator/4
  Gain5/1 -> MATLAB Function/2(front_leftFront_uss_dist)
  Gain11/1 -> MATLAB Function/8(rear_leftRear_uss_dist)
  Gain4/1 -> MATLAB Function/1(front_leftSide_uss_dist)
  In13/1 -> MATLAB Function/13(USS_Position)
  gASI_u16FRObsDist/1 -> BusCreator/2
  Gain12/1 -> MATLAB Function/9(rear_leftMiddle_uss_dist)
  Gain8/1 -> MATLAB Function/5(front_rightFront_uss_dist)
  gASI_u16RRSideObsDist/1 -> BusCreator/12
  Gain14/1 -> MATLAB Function/11(rear_rightRear_uss_dist)
  Gain6/1 -> MATLAB Function/3(front_leftMiddle_uss_dist)
  gASI_u16RrtMidLObsDist/1 -> BusCreator/7
  Gain15/1 -> MATLAB Function/12(rear_rightSide_uss_dist)
  BusSelector/2 -> Gain5/1  "<gASI_u16FLObsDist>"
  BusSelector/7 -> Gain10/1  "<gASI_u16RLSideObsDist>"
  gASI_u16RLSideObsDist/1 -> BusCreator/11
  BusSelector/9 -> Gain12/1  "<gASI_u16RrtMidLObsDist>"
  gASI_u16FLSideObsDist/1 -> BusCreator/9
  gASI_u16RLObsDist/1 -> BusCreator/5
  gASI_u16RrtMidRObsDist/1 -> BusCreator/8
  gASI_u16FLObsDist/1 -> BusCreator/1
  gASI_u16FrtMidLObsDist/1 -> BusCreator/3
  Constant/1 -> Obj_Position_Identify/2(Err_USS)
  Constant1/1 -> Find_Obj_USS_ID/2(Blind_Err)
  Obj_Position_Identify/1(Aera_Case_flag) -> [Aera_Case_flag]
  Find_Obj_USS_ID/2(Detect_Sum) -> Goto2/1
  Find_Obj_USS_ID/1(Detection_ID) -> Goto1/1
  [Sensor_Detection] -> Obj_Position_Identify/1(Sensor_Detection)
  From4/1 -> Find_Obj_USS_ID/1(Sensor_Detection)
  [Sensor_Detection] -> BusSelector/1
  [Single_Switch] -> Detection Processment/1(In1)
  [Sensor_Detection] -> Detection Processment/2(In2)
  [Triangle_Switch] -> Detection Processment/3(In3)
  [Sensor_Detection] -> Detection Processment/4(In4)
  Detection Processment/3(Out3) -> [Obj_Triangle_USS_Lgtl]
  [Aera_Case_flag] -> State Switch/1(In1)
  State Switch/1(Out1) -> [Single_Switch]
  State Switch/2(Out2) -> [Triangle_Switch]
  Detection Processment/2(Out2) -> [Obj_Single_USS_Latl]
  Detection Processment/4(Out4) -> [Obj_Triangle_USS_Latl]
  Detection Processment/1(Out1) -> [Obj_Single_USS_Lgtl]
  [Obj_Single_USS_Lgtl] -> Out6/1
  [Obj_Single_USS_Latl] -> Out1/1
  [Obj_Triangle_USS_Lgtl] -> Out2/1
  [Obj_Triangle_USS_Latl] -> Out3/1
  State Switch/3(Out3) -> Terminator/1
  [Aera_Case_flag] -> Out4/1
  Data Type Conversion/1 -> [Sensor_Detection]

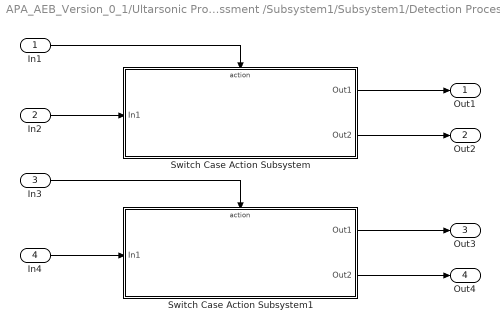
== system APA_AEB_Version_0_1/Ultarsonic Processment /Subsystem1/Subsystem1/Detection Processment ==
  In1 : Inport
  In2 : Inport  Port=2
  In3 : Inport  Port=3
  In4 : Inport  Port=4
  Switch Case Action Subsystem : Subsystem  TreatAsAtomicUnit=on
  Switch Case Action Subsystem1 : Subsystem  TreatAsAtomicUnit=on
  Out1 : Outport
  Out2 : Outport  Port=2
  Out3 : Outport  Port=3
  Out4 : Outport  Port=4
  wires:
  In3/1 -> Switch Case Action Subsystem1/Action
  In4/1 -> Switch Case Action Subsystem1/1(In1)
  In1/1 -> Switch Case Action Subsystem/Action
  Switch Case Action Subsystem1/1(Out1) -> Out3/1
  In2/1 -> Switch Case Action Subsystem/1(In1)
  Switch Case Action Subsystem/1(Out1) -> Out1/1
  Switch Case Action Subsystem/2(Out2) -> Out2/1
  Switch Case Action Subsystem1/2(Out2) -> Out4/1

== system APA_AEB_Version_0_1/Ultarsonic Processment /Subsystem1/Subsystem1/State Switch ==
  In1 : Inport
  Switch Case : SwitchCase  CaseConditions={[1,2,3,4,5,6,7,8,9,10,11,12],[14,15,16,20,21,22]}
  Out1 : Outport
  Out2 : Outport  Port=2
  Out3 : Outport  Port=3
  wires:
  Switch Case/3 -> Out3/1
  In1/1 -> Switch Case/1
  Switch Case/2 -> Out2/1
  Switch Case/1 -> Out1/1

== system APA_AEB_Version_0_1/Ultarsonic Processment /Subsystem1/Subsystem1/Detection Processment/Switch Case Action Subsystem ==
  In1 : Inport
  Action Port : ActionPort  ActionPortLabel=case [ 1 2 3 4 5 6 7 8 9 10 11 12 ]:
  MATLAB Function : MATLAB Function  TreatAsAtomicUnit=on
  Out1 : Outport
  Out2 : Outport  Port=2
  wires:
  In1/1 -> MATLAB Function/1(Sensor_Detection)
  MATLAB Function/1(Longitudial_Dist) -> Out1/1
  MATLAB Function/2(Lateral_Dist) -> Out2/1

== system APA_AEB_Version_0_1/Ultarsonic Processment /Subsystem1/Subsystem1/Detection Processment/Switch Case Action Subsystem1 ==
  In1 : Inport
  Action Port : ActionPort  ActionPortLabel=case [ 14 15 16 20 21 22 ]:
  MATLAB Function : MATLAB Function  TreatAsAtomicUnit=on
  Out1 : Outport
  Out2 : Outport  Port=2
  wires:
  In1/1 -> MATLAB Function/1(Sensor_Detection)
  MATLAB Function/1(Longitudial_triDist) -> Out1/1
  MATLAB Function/2(Lateral_triDist) -> Out2/1

== matlab function APA_AEB_Version_0_1/Vehicle Prediction/Subsystem/Foward Brake Distance Calculation ==
  data: Vehicle_Speed_NonDriven input single; Brake_Dist output single
function Brake_Dist = Fowward_Brake_Dist_Cal(Vehicle_Speed_NonDriven)
% 计算不同车速下的制动距离 
% Brake_Dist: 所需的制动距离
% Vehicle_Speed_NonDriven: 当时的车速
p1 =        5.43;
p2 =       -10.5;
p3 =       9.452;
p4 =     -0.8946;

Brake_Dist = p1*Vehicle_Speed_NonDriven^3 + p2*Vehicle_Speed_NonDriven^2 + p3*Vehicle_Speed_NonDriven + p4;

== matlab function APA_AEB_Version_0_1/Vehicle Prediction/Subsystem1/Steer Angle To Wheel Angle ==
  data: Steer_Angle input single; Wheel_Angle output single
function Wheel_Angle = StrAngle_To_WheelAngle(Steer_Angle)
% 计算不同方向盘转角对应的轮胎转角
% Wheel_Angle: 车轮转角
% Steer_Angle: 方向盘转角
p1 =  -2.194e-18;
p2 =   1.258e-15;
p3 =  -1.478e-14;
p4 =   2.125e-10;
p5 =  -1.838e-07;
p6 =    0.001145;
p7 =   -0.001468; 

Wheel_Angle = p1*Steer_Angle^6 + p2*Steer_Angle^5 + p3*Steer_Angle^4 + p4*Steer_Angle^3 + p5*Steer_Angle^2 + p6*Steer_Angle + p7;

== matlab function APA_AEB_Version_0_1/Vehicle Prediction/Subsystem/Backward Brake Distance Calculation ==
  data: Vehicle_Speed_NonDriven input single; Brake_Dist output single
function Brake_Dist = Backward_Brake_Dist_Cal(Vehicle_Speed_NonDriven)
% 计算不同车速下的制动距离 
% Brake_Dist: 所需的制动距离
% Vehicle_Speed_NonDriven: 当时的车速
p1 =        5.43;
p2 =       -10.5;
p3 =       9.452;
p4 =     -0.8946;

Brake_Dist = p1*Vehicle_Speed_NonDriven^3 + p2*Vehicle_Speed_NonDriven^2 + p3*Vehicle_Speed_NonDriven + p4;

== matlab function APA_AEB_Version_0_1/Translate Sensor Position to Distance ==
  data: USS_Position input single; USS_Dist output single
function USS_Dist= USS_MountPos_Translation(USS_Position)
% 计算相邻两个超声波雷达之间的距离

USS_Dist_1_2 = single(norm(USS_Position(1,:) - USS_Position(2,:)));
USS_Dist_2_3 = single(norm(USS_Position(2,:) - USS_Position(3,:)));
USS_Dist_3_4 = single(norm(USS_Position(3,:) - USS_Position(4,:)));
USS_Dist_4_5 = single(norm(USS_Position(4,:) - USS_Position(5,:)));
USS_Dist_5_6 = single(norm(USS_Position(5,:) - USS_Position(6,:)));
USS_Dist_6_7 = single(norm(USS_Position(6,:) - USS_Position(7,:)));
USS_Dist_7_8 = single(norm(USS_Position(7,:) - USS_Position(8,:)));
USS_Dist_8_9 = single(norm(USS_Position(8,:) - USS_Position(9,:)));
USS_Dist_9_10 = single(norm(USS_Position(9,:) - USS_Position(10,:)));
USS_Dist_10_11 = single(norm(USS_Position(10,:) - USS_Position(11,:)));
USS_Dist_11_12 = single(norm(USS_Position(11,:) - USS_Position(12,:)));
USS_Dist_1_12 = single(norm(USS_Position(1,:) - USS_Position(12,:)));

% USS_Dist.USS_Dist_1_2 = USS_Dist_1_2;
% USS_Dist.USS_Dist_2_3 = USS_Dist_2_3;
% USS_Dist.USS_Dist_2_3 = USS_Dist_2_3;
USS_Dist = [USS_Dist_1_2 USS_Dist_2_3 USS_Dist_3_4 USS_Dist_4_5 USS_Dist_5_6 USS_Dist_6_7 USS_Dist_7_8 USS_Dist_8_9 USS_Dist_9_10 USS_Dist_10_11 USS_Dist_11_12 USS_Dist_1_12];
